simulink model "slexPrinterExample_org"  (Simulink 10.0)
settings: Solver=FixedStepDiscrete  StartTime=0.0  StopTime=200  RelTol=1e-3  EnableMultiTasking=on
model workspace (MATLAB code in the model file):
  | INK_MIN=1;
  | PRINT_RATE=1;
undefined symbols (not defined in the file): job, queuePrintJob
settings Model: Creator=The MathWorks, Inc.  ModifiedByFormat=The MathWorks Inc.  LastModifiedBy=The MathWorks Inc.  ExtModeAutoUpdateStatusClock=off
settings DataIOCC: LimitDataPoints=on  ReturnWorkspaceOutputs=on  SignalLoggingName=sigsOut
settings OptimizationCC: ExpressionDepthLimit=2147483647  InitFltsAndDblsToZero=on  EfficientMapNaN2IntZero=off  LifeSpan=Inf  EfficientTunableParamExpr=on
settings DebuggingCC: SaveWithParameterizedLinksMsg=none  UnderspecifiedInitializationDetection=Simplified  MergeDetectMultiDrivingBlocksExec=error  SignalResolutionControl=TryResolveAllWithWarning  BlockPriorityViolationMsg=error  AllowSymbolicDim=off  StateNameClashWarn=warning  PregeneratedLibrarySubsystemCodeDiagnostic=none
settings HardwareCC: TargetBitPerLong=64  TargetBitPerPointer=64  TargetBitPerSizeT=64  TargetBitPerPtrDiffT=64  TargetLongLongMode=on  TargetIntDivRoundTo=Zero  TargetEndianess=LittleEndian  TargetWordSize=64  TargetHWDeviceType=MATLAB Host  ProdEqTarget=off
settings SFSimCC: SFSimEcho=off  SimIntegrity=off  SimParseCustomCode=off  MATLABDynamicMemAlloc=off
settings RTWCC: Description=Real-Time Workshop Embedded Coder  SystemTargetFile=ert.tlc  TemplateMakefile=ert_default_tmf  GenerateReport=on  IncludeHyperlinkInReport=on  LaunchReport=on  GenerateTraceInfo=on  GenerateTraceReport=on  GenerateTraceReportSl=on  GenerateTraceReportSf=on  GenerateTraceReportEml=on
settings CodeAppCC: IgnoreCustomStorageClasses=off  CustomSymbolStrType=$N$R$M  InternalIdentifier=Classic
settings ERTTargetCC: MultiwordLength=2048  GenerateSampleERTMain=on  ERTCustomFileTemplate=example_file_process.tlc  ConvertIfToSwitch=off  SuppressUnreachableDefaultCases=off
settings ConfigComp: CovMetricSettings=dcmtr  CovShowResultsExplorer=off  CovExternalEMLEnable=off  CovSFcnEnable=off

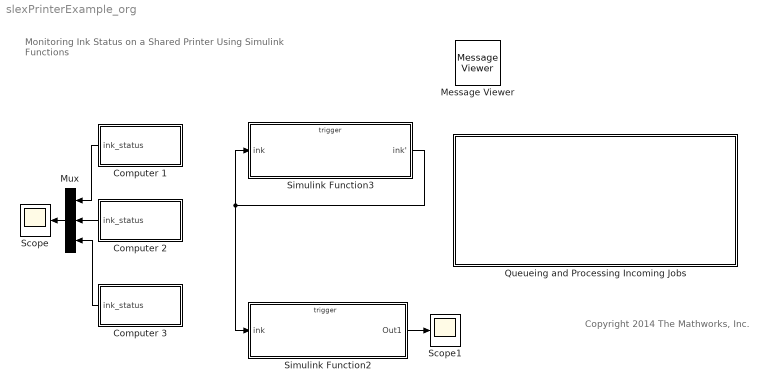
== system slexPrinterExample_org ==
  note: Monitoring Ink Status on a Shared Printer
      | Using Simulink Functions
  note: Copyright 2014 The Mathworks, Inc.
  Computer 1 : Subsystem  TreatAsAtomicUnit=on
  Computer 2 : Subsystem  TreatAsAtomicUnit=on
  Computer 3 : Subsystem  TreatAsAtomicUnit=on
  Message Viewer : MessageViewer  SavedRootId=#
  Mux : Mux  Inputs=3
  Queueing and Processing Incoming Jobs : Stateflow chart  TreatAsAtomicUnit=on
  Scope : Scope
  Scope1 : Scope
  Simulink Function2 : Subsystem  TreatAsAtomicUnit=on
  Simulink Function3 : Subsystem  TreatAsAtomicUnit=on
  wires:
  Simulink Function3/1(ink') -> Simulink Function2/1(ink), Simulink Function3/1(ink)
  Computer 1/1(ink_status) -> Mux/1
  Computer 2/1(ink_status) -> Mux/2
  Computer 3/1(ink_status) -> Mux/3
  Mux/1 -> Scope/1
  Simulink Function2/1(Out1) -> Scope1/1

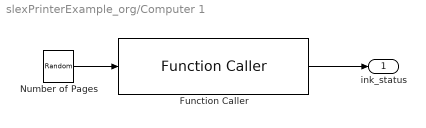
== system slexPrinterExample_org/Computer 1 ==
  Function Caller : FunctionCaller  FunctionPrototype=ink_status = addPrintJob(job)  InputArgumentSpecifications=<Enter example>  OutputArgumentSpecifications=<Enter example>
  Number of Pages : UniformRandomNumber  Minimum=0  Maximum=.5  SampleTime=1
  ink_status : Outport  VectorParamsAs1DForOutWhenUnconnected=off
  wires:
  Number of Pages/1 -> Function Caller/1
  Function Caller/1 -> ink_status/1

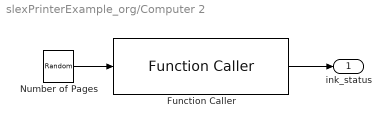
== system slexPrinterExample_org/Computer 2 ==
  Function Caller : FunctionCaller  FunctionPrototype=ink_status = addPrintJob(job)  InputArgumentSpecifications=<Enter example>  OutputArgumentSpecifications=<Enter example>
  Number of Pages : UniformRandomNumber  Minimum=0  Maximum=.5  SampleTime=1
  ink_status : Outport  InitialOutput=100  VectorParamsAs1DForOutWhenUnconnected=off
  wires:
  Number of Pages/1 -> Function Caller/1
  Function Caller/1 -> ink_status/1

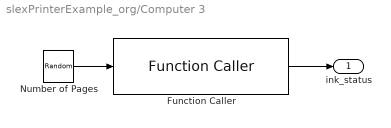
== system slexPrinterExample_org/Computer 3 ==
  Function Caller : FunctionCaller  FunctionPrototype=ink_status = addPrintJob(job)  InputArgumentSpecifications=<Enter example>  OutputArgumentSpecifications=<Enter example>
  Number of Pages : UniformRandomNumber  Minimum=0  Maximum=.5  SampleTime=1
  ink_status : Outport  InitialOutput=100  VectorParamsAs1DForOutWhenUnconnected=off
  wires:
  Number of Pages/1 -> Function Caller/1
  Function Caller/1 -> ink_status/1

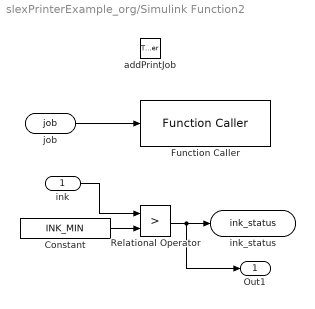
== system slexPrinterExample_org/Simulink Function2 ==
  ink : Inport
      settings: LatchInputForFeedbackSignals=on
  addPrintJob : TriggerPort  TriggerType=function-call  IsSimulinkFunction=on  FunctionName=addPrintJob  VariantControl=Variant
  Constant : Constant  Value=INK_MIN
  Function Caller : FunctionCaller  FunctionPrototype=queuePrintJob(job)  InputArgumentSpecifications=1  OutputArgumentSpecifications=<Enter example>
  Relational Operator : RelationalOperator  Operator=>  OutDataTypeStr=boolean  RndMeth=Nearest
  job : ArgIn  DisableCoverage=on  ArgumentName=job
  ink_status : ArgOut  OutDataTypeStr=boolean  ArgumentName=ink_status
  Out1 : Outport  VectorParamsAs1DForOutWhenUnconnected=off
  wires:
  job/1 -> Function Caller/1
  ink/1 -> Relational Operator/1
  Constant/1 -> Relational Operator/2
  Relational Operator/1 -> Out1/1, ink_status/1

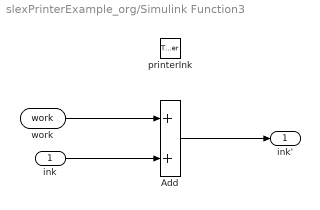
== system slexPrinterExample_org/Simulink Function3 ==
  ink : Inport
      settings: LatchInputForFeedbackSignals=on
  printerInk : TriggerPort  TriggerType=function-call  IsSimulinkFunction=on  FunctionName=printerInk  VariantControl=Variant
  Add : Sum
  work : ArgIn  DisableCoverage=on  ArgumentName=work
  ink' : Outport  InitialOutput=100  VectorParamsAs1DForOutWhenUnconnected=off
  wires:
  work/1 -> Add/1
  Add/1 -> ink'/1
  ink/1 -> Add/2

== stateflow chart Queueing and Processing Incoming Jobs ==
  settings: updateMethod=DISCRETE  sampleTime=1
  state Idle
  state queuePrintJob(job) [function]
    (default) -> (junction 7) : { work = work + job; }
  state Busy
    du:
    work = work-PRINT_RATE;
    printerInk(-PRINT_RATE);
  (default) -> Idle
  Idle -> Busy : [work > 0]
  Busy -> Idle : [work <= 0]
  data: job function_input double size=1; work local double; PRINT_RATE parameter double
